simulink model "second"  (R2023b)
settings: Solver=VariableStepAuto  StartTime=0.0  StopTime=5.0  RelTol=1e-3
values from neighbouring files (symbols this model uses):
  b = 0.05    [main.m]
  l = 0.3    [main.m]
  m = 0.2    [main.m]
settings Model: Creator=Егор  LastModifiedBy=Егор

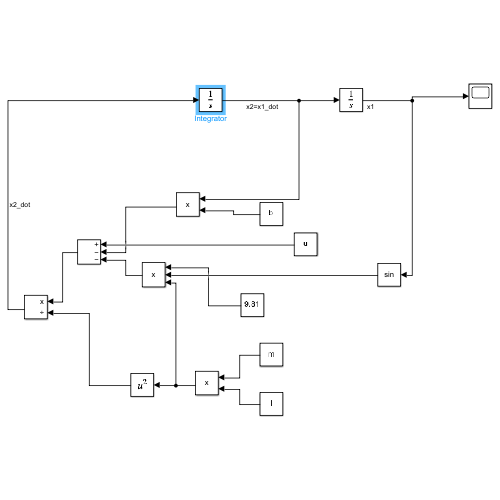
[thumbnail: Simulink's stored preview of the top-level diagram]
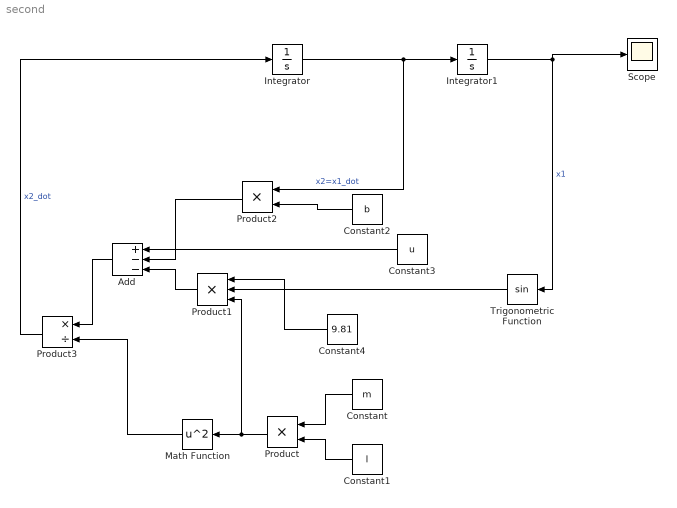
== system second ==
  Add : Sum  Inputs=+--
  Constant : Constant  Value=m
  Constant1 : Constant  Value=l
  Constant2 : Constant  Value=b
  Constant3 : Constant  Value=u
  Constant4 : Constant  Value=9.81
  Integrator : Integrator  InitialCondition=pi/4
  Integrator1 : Integrator
  Math Function : Math  Operator=square
  Product : Product
  Product1 : Product  Inputs=3
  Product2 : Product
  Product3 : Product  Inputs=*/
  Scope : Scope
  Trigonometric Function : Trigonometry
  wires:
  Integrator/1 -> Product2/1, Integrator1/1  "x2=x1_dot"
  Product3/1 -> Integrator/1  "x2_dot"
  Integrator1/1 -> Scope/1, Trigonometric Function/1  "x1"
  Constant/1 -> Product/1
  Constant1/1 -> Product/2
  Product/1 -> Product1/3, Math Function/1
  Trigonometric Function/1 -> Product1/2
  Constant4/1 -> Product1/1
  Product1/1 -> Add/3
  Constant2/1 -> Product2/2
  Constant3/1 -> Add/1
  Product2/1 -> Add/2
  Math Function/1 -> Product3/2
  Add/1 -> Product3/1
